simulink model "MAS_2021"  (R2023a)
settings: Solver=ode4  StartTime=0.0  StopTime=1  FixedStep=1e-6  RelTol=1e-6
values from neighbouring files (symbols this model uses):
  abc_alpha_beta = sqrt(2/3) * [1, -1/2, -1/2 ... (first row only)    [main.m]
  Flux_1 = 1/(Msr^2 - Ls * Lr )  * [Rs*Lr, 0, -Rs*Msr, 0 ... (first row only)    [main.m]
  Flux_2 = 1/(Msr^2 - Ls * Lr )  * [0, 0, 0, 0 ... (first row only)    [main.m]
  frot = 0.01    [main.m]
  In = 8.3    [main.m]
  Inv_abc_alpha_beta = inv(abc_alpha_beta)    [main.m]
  Inv_Phi_Courant = inv(Phi_Courant)    [main.m]
  J = 0.025    [main.m]
  K_reg_flux = (2*xi_reg_flux*wo_reg_flux*Lr/Rr-1)/Msr    [main.m]
  K_reg_vitesse = (2*xi_reg_vitesse*wo_reg_vitesse*T_meca-1)*frot    [main.m]
  ki = 2*wo_reg_courant*sigma*Ls*xi_reg-Rsr    [main.m]
  Kpi = ws*20    (= 6283.18530718)    [main.m]
  Lr = 0.194    [main.m]
  Ls = 0.182    [main.m]
  Msr = 0.182    [main.m]
  onduleur = V_MLI/3*[2,-1,-1 ... (first row only)    [main.m]
  p = 2    [main.m]
  Rr = 1.15    [main.m]
  sigma = 1-Msr^2/(Ls*Lr)    (= 0.0618556701031)    [main.m]
  T_charge = 0    [main.m]
  T_MLI = 1/F_MLI    (= 0.0001)    [main.m]
  T_reg_flux = Msr*K_reg_flux*Lr/(Rr*wo_reg_flux^2)    [main.m]
  T_reg_vitesse = K_reg_vitesse/(T_meca*frot*wo_reg_vitesse^2)    [main.m]
  Tfiltre = 1e-5    (= 1e-05)    [main.m]
  Ti = ki/(wo_reg_courant^2*Ls*sigma)    [main.m]
  Tin = sqrt(10)/Kpi    [main.m]
  Trau = T_meca*1e-3    (= 0.0025)    [main.m]
  V_MLI = 540    [main.m]
  Vn = 380    [main.m]
  ws = 2*pi*Fn    (= 314.159265359)    [main.m]
libraries: simulink_extras x6, hdlsllib x5, simulink x2
settings Model: SimulationMode=accelerator  Creator=philippecasteres  LastModifiedBy=philippecasteres
settings SolverCC: ZeroCrossAlgorithm=Adaptive
settings DebuggingCC: IgnoredZcDiagnostic=none

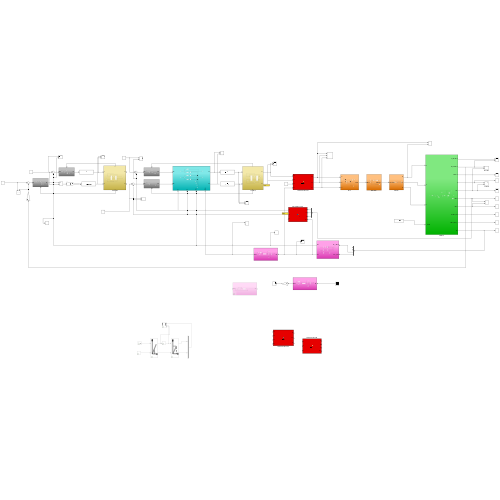
[thumbnail: Simulink's stored preview of the top-level diagram]
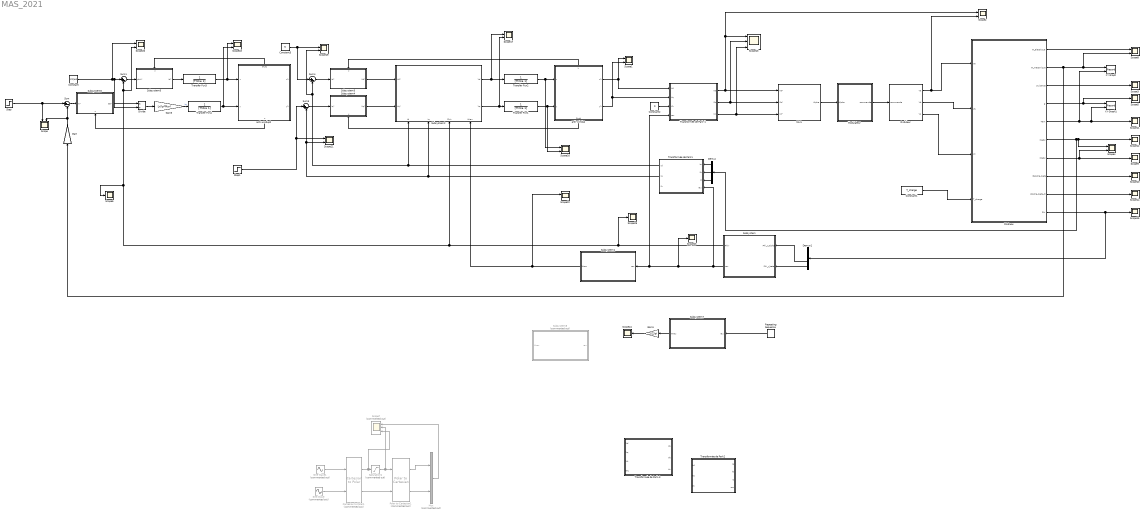
== system MAS_2021 ==
  Cartesian to Polar1 : simulink_extras/Transformations/Cartesian to Polar  Commented=on
  Constant : Constant  Value=Vn/ws
  Constant1 : Constant  Value=T_charge
  Constant2 : Constant  Value=0
  Constant3 : Constant  Value=5
  Demux : Demux  Outputs=3
  Demux1 : Demux
  Divide : Product  Inputs=*/
  Gain : Gain  Gain=30/pi
  Gain1 : Gain  Gain=1/2/pi
  Gain3 : Gain  Gain=Lr/(p*Msr)
  MASnew : Subsystem
  MLI1 : Subsystem
  Modulateur : Subsystem
  Mux : Mux  Commented=on  Inputs=2
  Onduleur : Subsystem
  Polar to Cartesian1 : simulink_extras/Transformations/Polar to Cartesian  Commented=on
  Repeating Sequence : simulink/Sources/Repeating Sequence  rep_seq_t=[0 1/100]  rep_seq_y=[0 2*pi]
  Saturation1 : Saturate  Commented=on  UpperLimit=215  LowerLimit=-sqrt(3/2)*Vn
  Scope{,1..2,4,8,16..22} (12 alike) : Scope  NumInputPorts=2
  Scope{3,5..6,9..12,14..15,23..25} (12 alike) : Scope
  Scope13 : Scope  NumInputPorts=3
  Scope7 : Scope  Commented=on  NumInputPorts=3
  Sine Wave : Sin  Commented=on  Amplitude=220  Frequency=50*2*pi  Phase=pi/2  SampleTime=0
  Sine Wave1 : Sin  Commented=on  Amplitude=220  Frequency=50*2*pi  SampleTime=0
  Step : Step  Time=0.1  After=1450  SampleTime=0
  Step1 : Step  Time=0.3  After=5  SampleTime=0
  Subsystem : Subsystem
  Subsystem1 : Subsystem
  Subsystem2 : Subsystem
      settings: PortSchema="{\"entries\":[{\"content\":{\"sides\":[{\"content\":{\"connectorIds\":[\"In1\",\"In2\"]},\"type\":\"ConnectorPlacement.EquallySpacedRectSide\",\"uuid\":\"374a3029-9c19-44eb-9b98-de55e62c7022\"},{\"content\":{\"connectorIds\":[\"Out1\",\"Out2\"],\"side\":\"RIGHT\"},\"type\":\"ConnectorPlacement.EquallySpacedRectSide\",\"uuid\":\"b066ba17-ce68-41f6-a300-7d3bc4dc3f92\"},{\"content\":{\"side\":\"TOP\"},\"type\":\"ConnectorPlacement.EquallySpacedRectSide\",\"uuid\":\"ed738241-ae45-464d-a05c-a5861c3f77ca\"},{\"content\":{\"connectorIds\":[\"In3\",\"In4\",\"In5\",\"In6\"],\"side\":\"BOTTOM\"},\"type\":\"ConnectorPlacement.EquallySpacedRectSide\",\"uuid\":\"e5249242-5c32-4682-b932-0c2aba441929\"}]},\"type\":\"ConnectorPlacement.EquallySpacedConnector\",\"uuid\":\"519ae50f-d565-4f6e-aabe-7acf3d791e4a\"}],\"packageUris\":[\"http://schema.mathworks.com/mf0/Connector/R2020b\"],\"version\":\"1.0\"}"
  Subsystem3 : Subsystem
      settings: PortSchema="{\"entries\":[{\"content\":{\"sides\":[{\"content\":{\"connectorIds\":[\"In1\"]},\"type\":\"ConnectorPlacement.EquallySpacedRectSide\",\"uuid\":\"e479fa30-fafe-4b33-9f29-bcdfd025492c\"},{\"content\":{\"connectorIds\":[\"Out1\"],\"side\":\"RIGHT\"},\"type\":\"ConnectorPlacement.EquallySpacedRectSide\",\"uuid\":\"004bb801-1125-495b-9383-1b89d3712869\"},{\"content\":{\"connectorIds\":[\"In2\"],\"side\":\"TOP\"},\"type\":\"ConnectorPlacement.EquallySpacedRectSide\",\"uuid\":\"eb300401-215a-493c-865f-c89d4f0da9de\"}]},\"type\":\"ConnectorPlacement.EquallySpacedConnector\",\"uuid\":\"4261b941-699b-4a50-9a10-aa37cbe6dd2a\"}],\"packageUris\":[\"http://schema.mathworks.com/mf0/Connector/R2020b\"],\"version\":\"1.0\"}"
  Subsystem4 : Subsystem
      settings: PortSchema="{\"entries\":[{\"content\":{\"sides\":[{\"content\":{\"connectorIds\":[\"In1\"]},\"type\":\"ConnectorPlacement.EquallySpacedRectSide\",\"uuid\":\"b47c6917-9341-4daa-88c1-000b41eb9d38\"},{\"content\":{\"connectorIds\":[\"Out1\"],\"side\":\"RIGHT\"},\"type\":\"ConnectorPlacement.EquallySpacedRectSide\",\"uuid\":\"db977880-8c33-40fc-933d-e73e745919fc\"},{\"content\":{\"side\":\"TOP\"},\"type\":\"ConnectorPlacement.EquallySpacedRectSide\",\"uuid\":\"c60e1241-7377-4c09-9831-21e7b95cd727\"},{\"content\":{\"connectorIds\":[\"In2\"],\"side\":\"BOTTOM\"},\"type\":\"ConnectorPlacement.EquallySpacedRectSide\",\"uuid\":\"7267beab-c733-40aa-ba5e-a945633c6122\"}]},\"type\":\"ConnectorPlacement.EquallySpacedConnector\",\"uuid\":\"e7c74c67-79e5-4b53-bf68-91e77d655faf\"}],\"packageUris\":[\"http://schema.mathworks.com/mf0/Connector/R2020b\"],\"version\":\"1.0\"}"
  Subsystem5 : Subsystem
      settings: PortSchema="{\"entries\":[{\"content\":{\"sides\":[{\"content\":{\"connectorIds\":[\"In1\"]},\"type\":\"ConnectorPlacement.EquallySpacedRectSide\",\"uuid\":\"b47c6917-9341-4daa-88c1-000b41eb9d38\"},{\"content\":{\"connectorIds\":[\"Out1\"],\"side\":\"RIGHT\"},\"type\":\"ConnectorPlacement.EquallySpacedRectSide\",\"uuid\":\"db977880-8c33-40fc-933d-e73e745919fc\"},{\"content\":{\"connectorIds\":[\"In2\"],\"side\":\"TOP\"},\"type\":\"ConnectorPlacement.EquallySpacedRectSide\",\"uuid\":\"c60e1241-7377-4c09-9831-21e7b95cd727\"}]},\"type\":\"ConnectorPlacement.EquallySpacedConnector\",\"uuid\":\"e7c74c67-79e5-4b53-bf68-91e77d655faf\"}],\"packageUris\":[\"http://schema.mathworks.com/mf0/Connector/R2020b\"],\"version\":\"1.0\"}"
  Subsystem6 : Subsystem
      settings: PortSchema="{\"entries\":[{\"content\":{\"sides\":[{\"content\":{\"connectorIds\":[\"In1\"]},\"type\":\"ConnectorPlacement.EquallySpacedRectSide\",\"uuid\":\"b47c6917-9341-4daa-88c1-000b41eb9d38\"},{\"content\":{\"connectorIds\":[\"Out1\"],\"side\":\"RIGHT\"},\"type\":\"ConnectorPlacement.EquallySpacedRectSide\",\"uuid\":\"db977880-8c33-40fc-933d-e73e745919fc\"},{\"content\":{\"side\":\"TOP\"},\"type\":\"ConnectorPlacement.EquallySpacedRectSide\",\"uuid\":\"c60e1241-7377-4c09-9831-21e7b95cd727\"},{\"content\":{\"connectorIds\":[\"In2\"],\"side\":\"BOTTOM\"},\"type\":\"ConnectorPlacement.EquallySpacedRectSide\",\"uuid\":\"995178c3-5227-47fa-849d-7fc8f375b837\"}]},\"type\":\"ConnectorPlacement.EquallySpacedConnector\",\"uuid\":\"e7c74c67-79e5-4b53-bf68-91e77d655faf\"}],\"packageUris\":[\"http://schema.mathworks.com/mf0/Connector/R2020b\"],\"version\":\"1.0\"}"
  Subsystem7 : Subsystem
  Subsystem8 : Subsystem  Commented=on
  Sum{,1,4..5} (4 alike) : Sum  Inputs=|+-
  Transfer Fcn{1..4} (4 alike) : TransferFcn  Denominator=[Tfiltre 1]
  Transformée de Park-1 : MATLAB Function  TreatAsAtomicUnit=on
  Transformée de Park-3 : MATLAB Function  TreatAsAtomicUnit=on
  Transformée de Park1 : MATLAB Function  TreatAsAtomicUnit=on
  Transformée de Park2 : MATLAB Function  TreatAsAtomicUnit=on
  XY Graph : Record  FileSettingsInternal="{\"entries\":[{\"content\":{\"excelSettings\":{\"content\":{},\"type\":\"Streamout.ExcelSettings\"}},\"type\":\"Streamout.FileSettingStorage\",\"uuid\":\"02bf0144-ef95-4ad2-a42f-d5bcd8c4972b\"}],\"packageUris\":[\"http://schema.mathworks.com/mf0/streamout_blocks/R2020a\"],\"version\":\"1.0\"}"  Layout=[1 1]  SignalsInternal="{\"entries\":[{\"content\":{\"signals\":[{\"content\":{\"blockPath\":[\"MAS_2021/XY Graph\"],\"dimensions\":[1],\"domain\":\"MAS_2021/XY Graph\",\"lineColor\":\"#a2142f\",\"plots\":[1],\"port\":1,\"sid\":[\"\"],\"signalID\":58272,\"signalName\":\"MASnew:2\"},\"type\":\"RecordBlkView.Signal\",\"uuid\":\"b78bae73-59df-4512-bf67-fe98b0d5a5c6\"},{\"content\":{\"blockPath\":[\"MAS_2021/XY Graph\"],\"dimensions\":[1],\"domain\":\"MAS_2021/XY Graph\",\"lineColor\":\"#139fff\",\"plots\":[1],\"port\":2,\"sid\":[\"\"],\"signalID\":58276,\"signalName\":\"MASnew:5\"},\"type\":\"RecordBlkView.Signal\",\"uuid\":\"1051b99f-fd16-496c-9762-0a6a3716ff38\"}]},\"type\":\"RecordBlkView.InputSignals\",\"uuid\":\"75fcb670-4d24-4ccf-8580-0be739766606\"}],\"packageUris\":[\"http://schema.mathworks.com/mf0/streamout_blocks/R2020a\"],\"version\":\"1.0\"}"  VisualizationBindings="{\"xyplotplugin\":{\"info\":[{\"series\":[{\"bindingParametersList\":[{\"parameter\":\"X-Axis\",\"signalID\":58272,\"signalName\":\"MASnew:2\"},{\"parameter\":\"Y-Axis\",\"signalID\":58276,\"signalName\":\"MASnew:5\"}],\"seriesID\":63116}],\"subplotID\":1}]}}"  CompatibilityTag=XY
  XY Graph1 : Record  FileSettingsInternal="{\"entries\":[{\"content\":{\"excelSettings\":{\"content\":{},\"type\":\"Streamout.ExcelSettings\"}},\"type\":\"Streamout.FileSettingStorage\",\"uuid\":\"62ad68df-1348-4f16-8d4f-e00fc3a6a313\"}],\"packageUris\":[\"http://schema.mathworks.com/mf0/streamout_blocks/R2020a\"],\"version\":\"1.0\"}"  Layout=[1 1]  SignalsInternal="{\"entries\":[{\"content\":{\"signals\":[{\"content\":{\"blockPath\":[\"MAS_2021/XY Graph1\"],\"dimensions\":[1],\"domain\":\"MAS_2021/XY Graph1\",\"lineColor\":\"#a2142f\",\"plots\":[1],\"port\":1,\"sid\":[\"\"],\"signalID\":58280,\"signalName\":\"MASnew:4\"},\"type\":\"RecordBlkView.Signal\",\"uuid\":\"248cccd2-926a-4347-ba54-2025f1e98270\"},{\"content\":{\"blockPath\":[\"MAS_2021/XY Graph1\"],\"dimensions\":[1],\"domain\":\"MAS_2021/XY Graph1\",\"lineColor\":\"#139fff\",\"plots\":[1],\"port\":2,\"sid\":[\"\"],\"signalID\":58284,\"signalName\":\"MASnew:5\"},\"type\":\"RecordBlkView.Signal\",\"uuid\":\"11fdf2ab-0bb6-4904-b875-f2617358f7f0\"}]},\"type\":\"RecordBlkView.InputSignals\",\"uuid\":\"8fda36b3-d89a-4054-b499-e537cb5cc1da\"}],\"packageUris\":[\"http://schema.mathworks.com/mf0/streamout_blocks/R2020a\"],\"version\":\"1.0\"}"  VisualizationBindings="{\"xyplotplugin\":{\"info\":[{\"series\":[{\"bindingParametersList\":[{\"parameter\":\"X-Axis\",\"signalID\":58280,\"signalName\":\"MASnew:4\"},{\"parameter\":\"Y-Axis\",\"signalID\":58284,\"signalName\":\"MASnew:5\"}],\"seriesID\":13282}],\"subplotID\":1}]}}"  CompatibilityTag=XY
  anti-windup : Subsystem
      settings: PortSchema="{\"entries\":[{\"content\":{\"sides\":[{\"content\":{\"connectorIds\":[\"In1\",\"In2\"]},\"type\":\"ConnectorPlacement.EquallySpacedRectSide\",\"uuid\":\"233cb3cb-1249-40bd-bfdc-45fa9814c46e\"},{\"content\":{\"connectorIds\":[\"Out1\",\"Out2\"],\"side\":\"RIGHT\"},\"type\":\"ConnectorPlacement.EquallySpacedRectSide\",\"uuid\":\"0fdc860d-9a1f-453b-acef-69f40f5c198e\"},{\"content\":{\"connectorIds\":[\"Out4\"],\"side\":\"TOP\"},\"type\":\"ConnectorPlacement.EquallySpacedRectSide\",\"uuid\":\"10667f9d-69ec-4f3a-8ac8-5b780339c6a9\"},{\"content\":{\"connectorIds\":[\"Out3\"],\"side\":\"BOTTOM\"},\"type\":\"ConnectorPlacement.EquallySpacedRectSide\",\"uuid\":\"5505156d-5de0-4527-aff8-81b020aef34d\"}]},\"type\":\"ConnectorPlacement.EquallySpacedConnector\",\"uuid\":\"a7d416d1-7b5f-49c4-ac6f-32e00a36b461\"}],\"packageUris\":[\"http://schema.mathworks.com/mf0/Connector/R2020b\"],\"version\":\"1.0\"}"
  anti-windup2 : Subsystem
      settings: PortSchema="{\"entries\":[{\"content\":{\"sides\":[{\"content\":{\"connectorIds\":[\"In1\",\"In2\"]},\"type\":\"ConnectorPlacement.EquallySpacedRectSide\",\"uuid\":\"233cb3cb-1249-40bd-bfdc-45fa9814c46e\"},{\"content\":{\"connectorIds\":[\"Out1\",\"Out2\"],\"side\":\"RIGHT\"},\"type\":\"ConnectorPlacement.EquallySpacedRectSide\",\"uuid\":\"0fdc860d-9a1f-453b-acef-69f40f5c198e\"},{\"content\":{\"connectorIds\":[\"Out4\"],\"side\":\"TOP\"},\"type\":\"ConnectorPlacement.EquallySpacedRectSide\",\"uuid\":\"10667f9d-69ec-4f3a-8ac8-5b780339c6a9\"},{\"content\":{\"connectorIds\":[\"Out3\"],\"side\":\"BOTTOM\"},\"type\":\"ConnectorPlacement.EquallySpacedRectSide\",\"uuid\":\"5505156d-5de0-4527-aff8-81b020aef34d\"}]},\"type\":\"ConnectorPlacement.EquallySpacedConnector\",\"uuid\":\"a7d416d1-7b5f-49c4-ac6f-32e00a36b461\"}],\"packageUris\":[\"http://schema.mathworks.com/mf0/Connector/R2020b\"],\"version\":\"1.0\"}"
  wires:
  Demux/1 -> Transformée de Park1/1(Ia)
  Demux/2 -> Transformée de Park1/2(Ib)
  Demux/3 -> Transformée de Park1/3(Ic)
  Constant1/1 -> MASnew/4(T_charge)
  Transformée de Park-1/2(Vb) -> MLI1/2(Vb*), Scope13/2
  Onduleur/1(Va) -> MASnew/1(Va), Scope2/2
  Transformée de Park-1/3(Vc) -> MLI1/3(Vc*), Scope13/3
  MASnew/8(ISalpha_beta) -> Scope10/1
  MASnew/3(puisance) -> Scope3/1
  MASnew/6(ISabc) -> Demux/1, Scope12/1, Scope4/1
  MASnew/7(IRabc) -> Scope4/2, Scope9/1
  Transformée de Park-1/1(Va) -> MLI1/1(Va*), Scope13/1, Scope2/1
  MASnew/2(W_mecanique) -> Scope8/2, XY Graph/1, Gain/1
  MASnew/1(W_electrique) -> Scope8/1
  MASnew/5(Tem) -> XY Graph/2, XY Graph1/2, Scope11/1
  MASnew/4(g) -> Scope5/1, XY Graph1/1
  MASnew/9(Valpha_beta_O) -> Scope14/1
  MASnew/10(Phi) -> Demux1/1, Scope15/1
  Onduleur/3(Vc) -> MASnew/3(Vc)
  Onduleur/2(Vb) -> MASnew/2(Vb)
  Sum4/1 -> Subsystem3/1(Id*)
  Transformée de Park1/1(Id) -> Subsystem2/3(Id), Sum4/2, Scope19/2
  Sum5/1 -> Subsystem4/1(Iq*)
  Subsystem5/1(Id*) -> Transfer Fcn3/1
  Gain3/1 -> Transfer Fcn4/1  "Iq"
  Transformée de Park1/2(Iq) -> Subsystem2/4(Iq), Scope21/2, Sum5/2
  Demux1/3 -> Subsystem/1(Phi_r_alpha)
  Demux1/4 -> Subsystem/2(Phi_r_beta)
  Subsystem/2(rau) -> Transformée de Park1/4(rau), Scope23/1, Subsystem1/1(rau), Transformée de Park-1/4(rau)
  Divide/1 -> Gain3/1
  Subsystem/1(Phir) -> Scope25/1, Subsystem2/5(Phir), Scope6/1, Scope20/2, Sum1/2
  Sum1/1 -> Subsystem5/1(phir*)
  Modulateur/1(commande) -> Onduleur/1(commande)
  MLI1/1(Alpha) -> Modulateur/1(Alpha)
  Constant/1 -> Scope20/1, Divide/2, Sum1/1
  Constant2/1 -> Transformée de Park-1/3(Vh)
  Step/1 -> Sum/1, Scope/1
  Gain/1 -> Scope/2, Sum/2
  Subsystem3/1(Vd*) -> Subsystem2/1(Vd*)
  Subsystem4/1(Vq*) -> Subsystem2/2(Vq*)
  Sum/1 -> Subsystem6/1(w*)
  Subsystem6/1(Ce*) -> Divide/1
  anti-windup2/3(u) -> Subsystem6/2(u)
  anti-windup2/4(Out1) -> Subsystem5/2(u)
  Cartesian to Polar1/2 -> Polar to Cartesian1/2
  Sine Wave/1 -> Cartesian to Polar1/2
  Sine Wave1/1 -> Cartesian to Polar1/1
  Polar to Cartesian1/1 -> Mux/1
  Polar to Cartesian1/2 -> Mux/2
  Mux/1 -> Scope7/1
  Saturation1/1 -> Scope7/2, Polar to Cartesian1/1
  Cartesian to Polar1/1 -> Scope7/3, Saturation1/1
  Subsystem2/2(Vq) -> Scope17/2, Transfer Fcn1/1
  anti-windup/4(u) -> Subsystem3/2(u)
  anti-windup/3(Out4) -> Subsystem4/2(u)
  Subsystem2/1(Vd) -> Scope17/1, Transfer Fcn2/1
  anti-windup/1(x1) -> Transformée de Park-1/1(Vd), Scope1/1
  anti-windup/2(y1) -> Transformée de Park-1/2(Vq), Scope1/2
  Transfer Fcn2/1 -> Scope16/1, anti-windup/1(x)
  Transfer Fcn1/1 -> Scope16/2, anti-windup/2(y)
  Transfer Fcn3/1 -> Scope18/1, anti-windup2/1(x)
  Transfer Fcn4/1 -> Scope18/2, anti-windup2/2(y)
  Constant3/1 -> Scope19/1, Sum4/1
  Step1/1 -> Sum5/1, Scope21/1
  Repeating Sequence/1 -> Subsystem7/1(rau)
  Subsystem7/1(Wrau) -> Gain1/1
  Gain1/1 -> Scope24/1
  Subsystem1/1(Wrau) -> Subsystem2/6(Wrau), Scope22/1

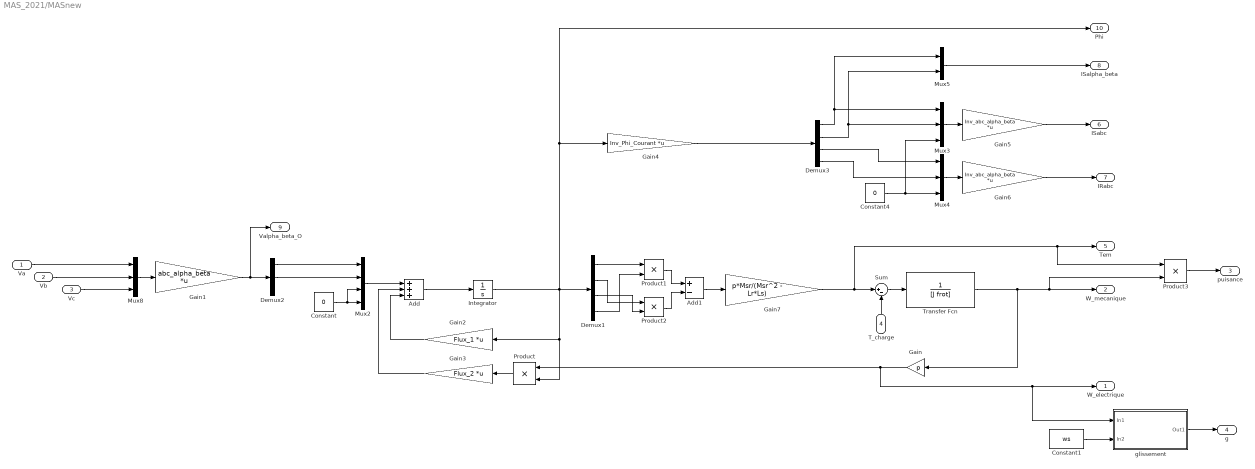
== system MAS_2021/MASnew ==
  Va : Inport
  Vb : Inport  Port=2
  Vc : Inport  Port=3
  T_charge : Inport  Port=4
  Add : Sum  Inputs=+++
  Add1 : Sum  Inputs=+-
  Constant : Constant  Value=0
  Constant1 : Constant  Value=ws
  Constant4 : Constant  Value=0
  Demux1 : Demux
  Demux2 : Demux  Outputs=3
  Demux3 : Demux
  Gain : Gain  Gain=p
  Gain1 : Gain  Gain=abc_alpha_beta  Multiplication=Matrix(K*u)
  Gain2 : Gain  Gain=Flux_1  Multiplication=Matrix(K*u)
  Gain3 : Gain  Gain=Flux_2  Multiplication=Matrix(K*u)
  Gain4 : Gain  Gain=Inv_Phi_Courant  Multiplication=Matrix(K*u)
  Gain5 : Gain  Gain=Inv_abc_alpha_beta  Multiplication=Matrix(K*u)
  Gain6 : Gain  Gain=Inv_abc_alpha_beta  Multiplication=Matrix(K*u)
  Gain7 : Gain  Gain=p*Msr/(Msr^2 - Lr*Ls)
  Integrator : Integrator
  Mux2 : Mux
  Mux3 : Mux  Inputs=3
  Mux4 : Mux  Inputs=3
  Mux5 : Mux  Inputs=2
  Mux8 : Mux  Inputs=3
  Product{,1..3} (4 alike) : Product
  Sum : Sum  Inputs=|+-
  Transfer Fcn : TransferFcn  Denominator=[J frot]
  glissement : Subsystem
  W_electrique : Outport
  W_mecanique : Outport  Port=2
  puisance : Outport  Port=3
  g : Outport  Port=4
  Tem : Outport  Port=5
  ISabc : Outport  Port=6
  IRabc : Outport  Port=7
  ISalpha_beta : Outport  Port=8
  Valpha_beta_O : Outport  Port=9
  Phi : Outport  Port=10
  wires:
  Demux3/4 -> Mux4/2
  Demux3/2 -> Mux3/2, Mux5/2
  T_charge/1 -> Sum/2
  Demux3/1 -> Mux3/1, Mux5/1
  Va/1 -> Mux8/1
  Sum/1 -> Transfer Fcn/1
  Demux1/1 -> Product1/1
  Demux3/3 -> Mux4/1
  Gain7/1 -> Sum/1, Product3/1, Tem/1
  Transfer Fcn/1 -> Gain/1, Product3/2, W_mecanique/1
  Add/1 -> Integrator/1
  Vc/1 -> Mux8/3
  Vb/1 -> Mux8/2
  Product/1 -> Gain3/1
  Integrator/1 -> Gain2/1, Product/2, Demux1/1, Gain4/1, Phi/1
  Mux2/1 -> Add/1
  Mux3/1 -> Gain5/1
  Mux5/1 -> ISalpha_beta/1
  Gain1/1 -> Valpha_beta_O/1, Demux2/1
  Mux8/1 -> Gain1/1
  Demux2/1 -> Mux2/1
  Demux2/2 -> Mux2/2
  Constant/1 -> Mux2/4, Mux2/3
  Gain2/1 -> Add/3
  Gain4/1 -> Demux3/1
  Constant4/1 -> Mux4/3, Mux3/3
  Gain5/1 -> ISabc/1
  Mux4/1 -> Gain6/1
  Gain6/1 -> IRabc/1
  Product1/1 -> Add1/1
  Product2/1 -> Add1/2
  Add1/1 -> Gain7/1
  Gain/1 -> glissement/1(In1), W_electrique/1, Product/1
  Gain3/1 -> Add/2
  Demux1/4 -> Product1/2
  Demux1/2 -> Product2/1
  Demux1/3 -> Product2/2
  Product3/1 -> puisance/1
  glissement/1(Out1) -> g/1
  Constant1/1 -> glissement/2(In2)

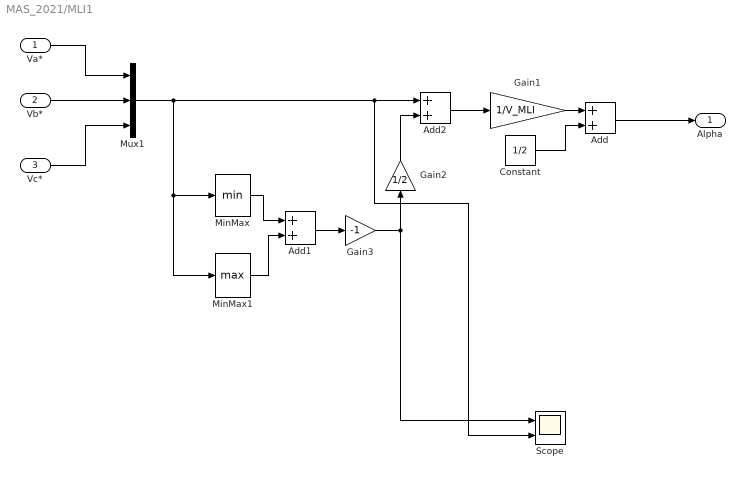
== system MAS_2021/MLI1 ==
  Va* : Inport
  Vb* : Inport  Port=2
  Vc* : Inport  Port=3
  Add : Sum
  Add1 : Sum
  Add2 : Sum
  Constant : Constant  Value=1/2
  Gain1 : Gain  Gain=1/V_MLI
  Gain2 : Gain  Gain=1/2
  Gain3 : Gain  Gain=-1
  MinMax : MinMax
  MinMax1 : MinMax  Function=max
  Mux1 : Mux  Inputs=3
  Scope : Scope  NumInputPorts=2
  Alpha : Outport
  wires:
  Va*/1 -> Mux1/1
  Gain1/1 -> Add/1
  Vb*/1 -> Mux1/2
  Vc*/1 -> Mux1/3
  Add/1 -> Alpha/1
  Add2/1 -> Gain1/1
  Constant/1 -> Add/2
  Gain2/1 -> Add2/2
  Mux1/1 -> Add2/1, Scope/2, MinMax/1, MinMax1/1
  Add1/1 -> Gain3/1
  MinMax/1 -> Add1/1
  MinMax1/1 -> Add1/2
  Gain3/1 -> Scope/1, Gain2/1

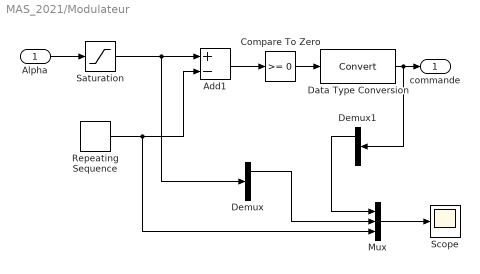
== system MAS_2021/Modulateur ==
  Alpha : Inport
  Add1 : Sum  Inputs=+-
  Compare To Zero : hdlsllib/Logic and Bit Operations/Compare To Zero  relop=>=  OutDataTypeStr=boolean
  Data Type Conversion : DataTypeConversion  SaturateOnIntegerOverflow=off  RndMeth=Floor
  Demux : Demux  Outputs=3
  Demux1 : Demux  Outputs=3
  Mux : Mux  Inputs=3
  Repeating Sequence : simulink/Sources/Repeating Sequence  rep_seq_t=[0 0.5*T_MLI T_MLI]  rep_seq_y=[1 0 1]
  Saturation : Saturate  UpperLimit=1  LowerLimit=0
  Scope : Scope
  commande : Outport
  wires:
  Alpha/1 -> Saturation/1
  Repeating Sequence/1 -> Mux/3, Add1/2
  Add1/1 -> Compare To Zero/1
  Saturation/1 -> Demux/1, Add1/1
  Compare To Zero/1 -> Data Type Conversion/1
  Data Type Conversion/1 -> Demux1/1, commande/1
  Mux/1 -> Scope/1
  Demux1/1 -> Mux/1
  Demux/1 -> Mux/2

== system MAS_2021/Onduleur ==
  commande : Inport
  Demux : Demux  Outputs=3
  Gain : Gain  Gain=onduleur  Multiplication=Matrix(K*u)
  Va : Outport
  Vb : Outport  Port=2
  Vc : Outport  Port=3
  wires:
  Gain/1 -> Demux/1
  commande/1 -> Gain/1
  Demux/3 -> Vc/1
  Demux/1 -> Va/1
  Demux/2 -> Vb/1

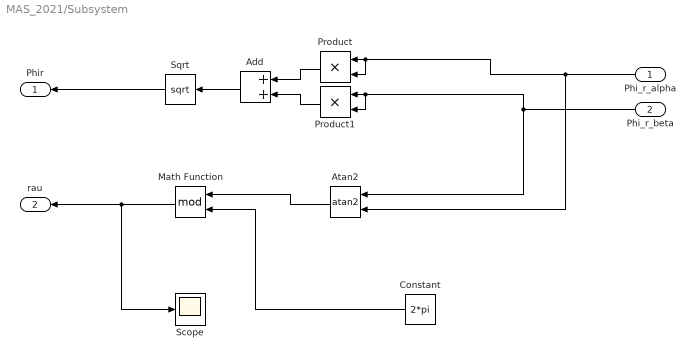
== system MAS_2021/Subsystem ==
  Phi_r_alpha : Inport
  Phi_r_beta : Inport  Port=2
  Add : Sum
  Atan2 : Trigonometry  Operator=atan2
  Constant : Constant  Value=2*pi
  Math Function : Math  Operator=mod
  Product : Product
  Product1 : Product
  Scope : Scope
  Sqrt : Sqrt
  Phir : Outport
  rau : Outport  Port=2
  wires:
  Sqrt/1 -> Phir/1
  Product1/1 -> Add/2
  Add/1 -> Sqrt/1
  Phi_r_beta/1 -> Atan2/1, Product1/2, Product1/1
  Product/1 -> Add/1
  Phi_r_alpha/1 -> Atan2/2, Product/2, Product/1
  Atan2/1 -> Math Function/1
  Constant/1 -> Math Function/2
  Math Function/1 -> Scope/1, rau/1

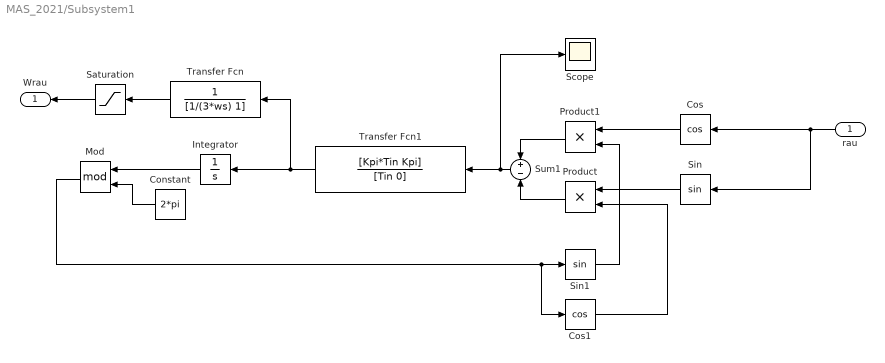
== system MAS_2021/Subsystem1 ==
  rau : Inport
  Constant : Constant  Value=2*pi
  Cos : Trigonometry  Operator=cos
  Cos1 : Trigonometry  Operator=cos
  Integrator : Integrator
  Mod : Math  Operator=mod
  Product : Product
  Product1 : Product
  Saturation : Saturate  UpperLimit=1.2*ws  LowerLimit=-1.2*ws
  Scope : Scope
  Sin : Trigonometry
  Sin1 : Trigonometry
  Sum1 : Sum  Inputs=+|-
  Transfer Fcn : TransferFcn  Denominator=[1/(3*ws) 1]
  Transfer Fcn1 : TransferFcn  Numerator=[Kpi*Tin Kpi]  Denominator=[Tin 0]
  Wrau : Outport
  wires:
  Constant/1 -> Mod/2
  Integrator/1 -> Mod/1
  Mod/1 -> Cos1/1, Sin1/1
  Sum1/1 -> Scope/1, Transfer Fcn1/1
  rau/1 -> Sin/1, Cos/1
  Sin/1 -> Product/1
  Cos/1 -> Product1/1
  Sin1/1 -> Product1/2
  Cos1/1 -> Product/2
  Product1/1 -> Sum1/1
  Product/1 -> Sum1/2
  Transfer Fcn/1 -> Saturation/1
  Transfer Fcn1/1 -> Transfer Fcn/1, Integrator/1
  Saturation/1 -> Wrau/1

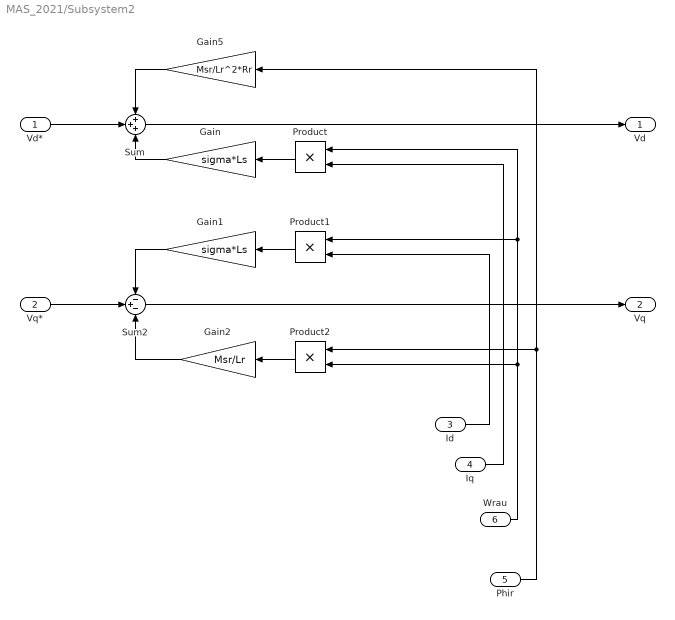
== system MAS_2021/Subsystem2 ==
  Vd* : Inport
  Vq* : Inport  Port=2
  Id : Inport  Port=3
  Iq : Inport  Port=4
  Phir : Inport  Port=5
  Wrau : Inport  Port=6
  Gain : Gain  Gain=sigma*Ls
  Gain1 : Gain  Gain=sigma*Ls
  Gain2 : Gain  Gain=Msr/Lr
  Gain5 : Gain  Gain=Msr/Lr^2*Rr
  Product : Product
  Product1 : Product
  Product2 : Product
  Sum : Sum  Inputs=+++
  Sum2 : Sum  Inputs=-+-
  Vd : Outport
  Vq : Outport  Port=2
  wires:
  Vd*/1 -> Sum/2
  Iq/1 -> Product/2
  Id/1 -> Product1/2
  Gain/1 -> Sum/3
  Product/1 -> Gain/1
  Gain1/1 -> Sum2/1
  Product1/1 -> Gain1/1
  Vq*/1 -> Sum2/2
  Wrau/1 -> Product2/2, Product1/1, Product/1
  Phir/1 -> Product2/1, Gain5/1
  Gain5/1 -> Sum/1
  Sum2/1 -> Vq/1
  Product2/1 -> Gain2/1
  Sum/1 -> Vd/1
  Gain2/1 -> Sum2/3

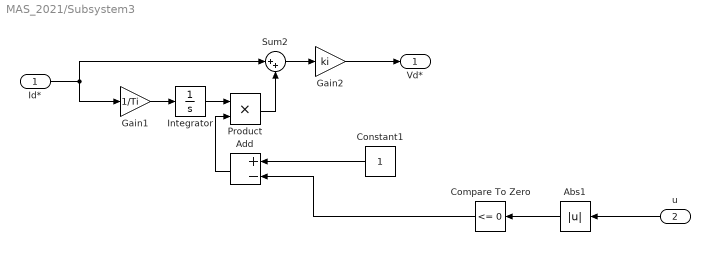
== system MAS_2021/Subsystem3 ==
  Id* : Inport
  u : Inport  Port=2
  Abs1 : Abs  SaturateOnIntegerOverflow=off
  Add : Sum  Inputs=+-
  Compare To Zero : hdlsllib/Logic and Bit Operations/Compare To Zero  relop=<=  OutDataTypeStr=boolean
  Constant1 : Constant
  Gain1 : Gain  Gain=1/Ti
  Gain2 : Gain  Gain=ki
  Integrator : Integrator
  Product : Product
  Sum2 : Sum  Inputs=|++
  Vd* : Outport
  wires:
  Gain1/1 -> Integrator/1
  Integrator/1 -> Product/1
  Add/1 -> Product/2
  Sum2/1 -> Gain2/1
  Id*/1 -> Gain1/1, Sum2/1
  Product/1 -> Sum2/2
  Gain2/1 -> Vd*/1
  Compare To Zero/1 -> Add/2
  Constant1/1 -> Add/1
  u/1 -> Abs1/1
  Abs1/1 -> Compare To Zero/1

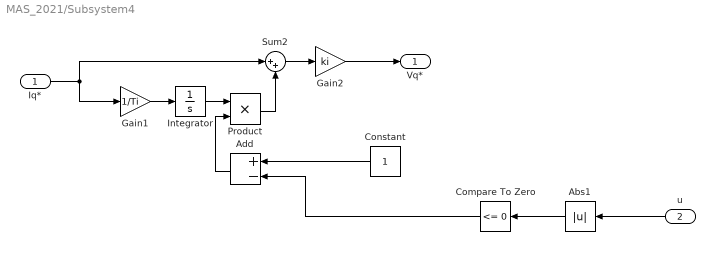
== system MAS_2021/Subsystem4 ==
  Iq* : Inport
  u : Inport  Port=2
  Abs1 : Abs  SaturateOnIntegerOverflow=off
  Add : Sum  Inputs=+-
  Compare To Zero : hdlsllib/Logic and Bit Operations/Compare To Zero  relop=<=  OutDataTypeStr=boolean
  Constant : Constant
  Gain1 : Gain  Gain=1/Ti
  Gain2 : Gain  Gain=ki
  Integrator : Integrator
  Product : Product
  Sum2 : Sum  Inputs=|++
  Vq* : Outport
  wires:
  Gain1/1 -> Integrator/1
  Integrator/1 -> Product/1
  Sum2/1 -> Gain2/1
  Iq*/1 -> Gain1/1, Sum2/1
  Product/1 -> Sum2/2
  Gain2/1 -> Vq*/1
  Constant/1 -> Add/1
  Add/1 -> Product/2
  Abs1/1 -> Compare To Zero/1
  u/1 -> Abs1/1
  Compare To Zero/1 -> Add/2

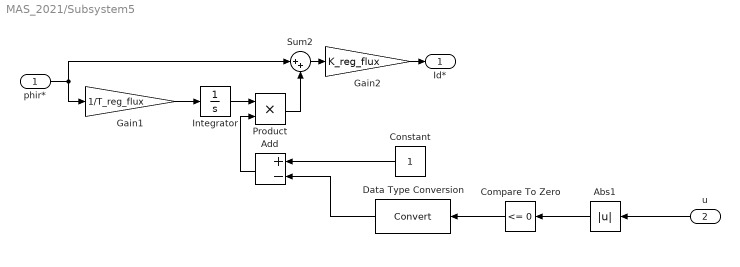
== system MAS_2021/Subsystem5 ==
  phir* : Inport
  u : Inport  Port=2
  Abs1 : Abs  SaturateOnIntegerOverflow=off
  Add : Sum  Inputs=+-
  Compare To Zero : hdlsllib/Logic and Bit Operations/Compare To Zero  relop=<=  OutDataTypeStr=boolean
  Constant : Constant
  Data Type Conversion : DataTypeConversion  SaturateOnIntegerOverflow=off  RndMeth=Floor
  Gain1 : Gain  Gain=1/T_reg_flux
  Gain2 : Gain  Gain=K_reg_flux
  Integrator : Integrator
  Product : Product
  Sum2 : Sum  Inputs=|++
  Id* : Outport
  wires:
  Gain1/1 -> Integrator/1
  Integrator/1 -> Product/1
  Add/1 -> Product/2
  Sum2/1 -> Gain2/1
  phir*/1 -> Sum2/1, Gain1/1
  Product/1 -> Sum2/2
  Gain2/1 -> Id*/1
  Constant/1 -> Add/1
  Data Type Conversion/1 -> Add/2
  Compare To Zero/1 -> Data Type Conversion/1
  Abs1/1 -> Compare To Zero/1
  u/1 -> Abs1/1

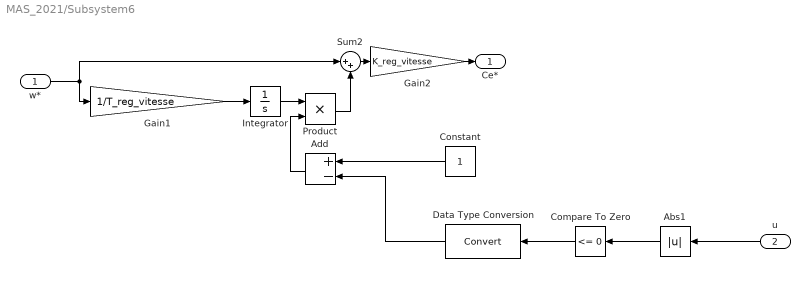
== system MAS_2021/Subsystem6 ==
  w* : Inport
  u : Inport  Port=2
  Abs1 : Abs  SaturateOnIntegerOverflow=off
  Add : Sum  Inputs=+-
  Compare To Zero : hdlsllib/Logic and Bit Operations/Compare To Zero  relop=<=  OutDataTypeStr=boolean
  Constant : Constant
  Data Type Conversion : DataTypeConversion  SaturateOnIntegerOverflow=off  RndMeth=Floor
  Gain1 : Gain  Gain=1/T_reg_vitesse
  Gain2 : Gain  Gain=K_reg_vitesse
  Integrator : Integrator
  Product : Product
  Sum2 : Sum  Inputs=|++
  Ce* : Outport
  wires:
  Gain1/1 -> Integrator/1
  Integrator/1 -> Product/1
  Sum2/1 -> Gain2/1
  w*/1 -> Gain1/1, Sum2/1
  Product/1 -> Sum2/2
  Gain2/1 -> Ce*/1
  Constant/1 -> Add/1
  Add/1 -> Product/2
  Data Type Conversion/1 -> Add/2
  Compare To Zero/1 -> Data Type Conversion/1
  Abs1/1 -> Compare To Zero/1
  u/1 -> Abs1/1

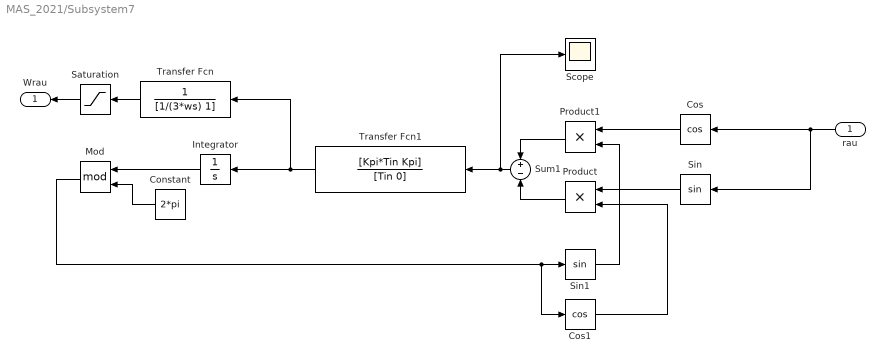
== system MAS_2021/Subsystem7 ==
  rau : Inport
  Constant : Constant  Value=2*pi
  Cos : Trigonometry  Operator=cos
  Cos1 : Trigonometry  Operator=cos
  Integrator : Integrator
  Mod : Math  Operator=mod
  Product : Product
  Product1 : Product
  Saturation : Saturate  UpperLimit=1.2*ws  LowerLimit=-1.2*ws
  Scope : Scope
  Sin : Trigonometry
  Sin1 : Trigonometry
  Sum1 : Sum  Inputs=+|-
  Transfer Fcn : TransferFcn  Denominator=[1/(3*ws) 1]
  Transfer Fcn1 : TransferFcn  Numerator=[Kpi*Tin Kpi]  Denominator=[Tin 0]
  Wrau : Outport
  wires:
  Constant/1 -> Mod/2
  Integrator/1 -> Mod/1
  Mod/1 -> Cos1/1, Sin1/1
  Sum1/1 -> Scope/1, Transfer Fcn1/1
  rau/1 -> Sin/1, Cos/1
  Sin/1 -> Product/1
  Cos/1 -> Product1/1
  Sin1/1 -> Product1/2
  Cos1/1 -> Product/2
  Product1/1 -> Sum1/1
  Product/1 -> Sum1/2
  Transfer Fcn/1 -> Saturation/1
  Transfer Fcn1/1 -> Transfer Fcn/1, Integrator/1
  Saturation/1 -> Wrau/1

== system MAS_2021/Subsystem8 ==
  rau : Inport
  Constant : Constant  Value=2*pi
  Integrator : Integrator
  Mod : Math  Operator=mod
  Sum6 : Sum  Inputs=|+-
  Transfer Fcn1 : TransferFcn  Denominator=[Trau 1]
  Wrau : Outport
  wires:
  Constant/1 -> Mod/2
  Integrator/1 -> Mod/1
  Mod/1 -> Sum6/2
  Transfer Fcn1/1 -> Wrau/1, Integrator/1
  rau/1 -> Sum6/1
  Sum6/1 -> Transfer Fcn1/1

== system MAS_2021/anti-windup ==
  x : Inport
  y : Inport  Port=2
  Cartesian to Polar : simulink_extras/Transformations/Cartesian to Polar
  Polar to Cartesian : simulink_extras/Transformations/Polar to Cartesian
  Saturation4 : Saturate  UpperLimit=V_MLI/sqrt(3)  LowerLimit=0
  Sum2 : Sum  Inputs=+|-
  Sum3 : Sum  Inputs=+|-
  x1 : Outport
  y1 : Outport  Port=2
  Out4 : Outport  Port=3
  u : Outport  Port=4
  wires:
  Polar to Cartesian/2 -> Sum3/2, y1/1
  Polar to Cartesian/1 -> Sum2/2, x1/1
  x/1 -> Cartesian to Polar/1, Sum2/1
  Sum2/1 -> u/1
  y/1 -> Cartesian to Polar/2, Sum3/1
  Cartesian to Polar/1 -> Saturation4/1
  Saturation4/1 -> Polar to Cartesian/1
  Cartesian to Polar/2 -> Polar to Cartesian/2
  Sum3/1 -> Out4/1

== system MAS_2021/anti-windup2 ==
  x : Inport
  y : Inport  Port=2
  Cartesian to Polar : simulink_extras/Transformations/Cartesian to Polar
  Polar to Cartesian : simulink_extras/Transformations/Polar to Cartesian
  Saturation4 : Saturate  UpperLimit=1.15*In  LowerLimit=0
  Sum2 : Sum  Inputs=+|-
  Sum3 : Sum  Inputs=+|-
  x1 : Outport
  y1 : Outport  Port=2
  u : Outport  Port=3
  Out1 : Outport  Port=4
  wires:
  Polar to Cartesian/2 -> y1/1, Sum3/2
  Polar to Cartesian/1 -> x1/1, Sum2/2
  x/1 -> Cartesian to Polar/1, Sum2/1
  Sum2/1 -> Out1/1
  y/1 -> Cartesian to Polar/2, Sum3/1
  Cartesian to Polar/1 -> Saturation4/1
  Saturation4/1 -> Polar to Cartesian/1
  Cartesian to Polar/2 -> Polar to Cartesian/2
  Sum3/1 -> u/1

== system MAS_2021/MASnew/glissement ==
  In1 : Inport
  In2 : Inport  Port=2
  Add2 : Sum  Inputs=+-
  Divide : Product  Inputs=*/
  Out1 : Outport
  wires:
  In2/1 -> Divide/2, Add2/1
  Divide/1 -> Out1/1
  In1/1 -> Add2/2
  Add2/1 -> Divide/1

== matlab function MAS_2021/Transformée de Park-1 ==
  data: Vd input; Va output; Vb output; Vc output; Vq input; Vh input; rau input
function [Va, Vb, Vc] = dq_abc(Vd,Vq,Vh,rau)


    % Vecteur de tensions d'entrée
    V = [Vd;Vq;Vh];
    
    % Matrice de transformation
    transformation_matrix = sqrt(2/3)*[cos(rau), cos(rau - 2*pi/3), cos(rau + 2*pi/3);
                                         -sin(rau), -sin(rau - 2*pi/3), -sin(rau + 2*pi/3);
                                          1/sqrt(2), 1/sqrt(2), 1/sqrt(2)];
    
    % Calcul des résultats
    result = inv(transformation_matrix) * V;
    
    % Attribution des résultats aux sorties
    Va = result(1);
    Vb= result(2);
    Vc = result(3);




end

== matlab function MAS_2021/Transformée de Park1 ==
  data: Ia input; Id output; Iq output; Ih output; Ib input; Ic input; rau input
function [Id,Iq,Ih] = abc_dq(Ia, Ib, Ic,rau)


    % Vecteur de tensions d'entrée
    I = [Ia; Ib; Ic];
    
    % Matrice de transformation
    transformation_matrix =sqrt(2/3)*[cos(rau), cos(rau - 2*pi/3), cos(rau + 2*pi/3);
                                         -sin(rau), -sin(rau - 2*pi/3), -sin(rau + 2*pi/3);
                                          1/sqrt(2), 1/sqrt(2), 1/sqrt(2)];
    
    % Calcul des résultats
    result = transformation_matrix * I;
    
    % Attribution des résultats aux sorties
    Id = result(1);
    Iq= result(2);
    Ih = result(3);




end

== matlab function MAS_2021/Transformée de Park-3 ==
  data: Vd input; Va output; Vb output; Vc output; Vq input; Vh input; rau input
function [Va, Vb, Vc] = dq_abc(Vd,Vq,Vh,rau)


    % Vecteur de tensions d'entrée
    V = [Vd;Vq;Vh];
    
    % Matrice de transformation
    transformation_matrix = sqrt(2/3)*[cos(rau), cos(rau - 2*pi/3), cos(rau + 2*pi/3);
                                         -sin(rau), -sin(rau - 2*pi/3), -sin(rau + 2*pi/3);
                                          1/sqrt(2), 1/sqrt(2), 1/sqrt(2)];
    
    % Calcul des résultats
    result = inv(transformation_matrix) * V;
    
    % Attribution des résultats aux sorties
    Va = result(1);
    Vb= result(2);
    Vc = result(3);




end

== matlab function MAS_2021/Transformée de Park2 ==
  data: Ia input; Id output; Iq output; Ih output; Ib input; Ic input; rau input
function [Id,Iq,Ih] = abc_dq(Ia, Ib, Ic,rau)


    % Vecteur de tensions d'entrée
    I = [Ia; Ib; Ic];
    
    % Matrice de transformation
    transformation_matrix = 2/3*[cos(rau), cos(rau - 2*pi/3), cos(rau + 2*pi/3);
                                         -sin(rau), -sin(rau - 2*pi/3), -sin(rau + 2*pi/3);
                                         1/2, 1/2, 1/2];
    
    % Calcul des résultats
    result = transformation_matrix * I;
    
    % Attribution des résultats aux sorties
    Id = result(1);
    Iq= result(2);
    Ih = result(3);




end
